simulink model "exemplo_bloco_Main"  (R2024b)
settings: Solver=ode45  StartTime=0.0  StopTime=200  RelTol=1e-6  EnableMultiTasking=on
settings Model: Creator=Mauricio  LastModifiedBy=johne
settings SolverCC: AlgebraicLoopSolver=TrustRegion
settings DataIOCC: LimitDataPoints=on  SaveFormat=Array  ReturnWorkspaceOutputs=off
settings OptimizationCC: LifeSpan=inf
settings DebuggingCC: SolverPrmCheckMsg=warning  UnconnectedInputMsg=warning  UnconnectedOutputMsg=warning  UnconnectedLineMsg=warning  SFUnexpectedBacktrackingDiag=warning  SFNoUnconditionalDefaultTransitionDiag=warning  SFExecutionAtInitializationDiag=none  ArithmeticOperatorsInVariantConditions=warning
settings HardwareCC: ProdBitPerPointer=32  ProdBitPerSizeT=32  ProdBitPerPtrDiffT=32  ProdLargestAtomicFloat=None  ProdIntDivRoundTo=Undefined  ProdEndianess=Unspecified  ProdWordSize=32  ProdHWDeviceType=32-bit Generic
settings ModelReferenceCC: EnableRefExpFcnMdlSchedulingChecks=on  PropagateSignalLabelsOutOfModel=off
settings SFSimCC: SimUseLocalCustomCode=off  CustomCodeUndefinedFunction=UseInterfaceOnly
settings RTWCC: RTWUseLocalCustomCode=off  GPUComputeCapability=3.5
settings CodeAppCC: StateflowObjectComments=on
settings GRTTargetCC: TargetLangStandard=C89/C90 (ANSI)
settings ConfigComp: CovMetricSettings=dw  CovSaveCumulativeToWorkspaceVar=on  CovSaveSingleToWorkspaceVar=on  CovExternalEMLEnable=off  CovSFcnEnable=off

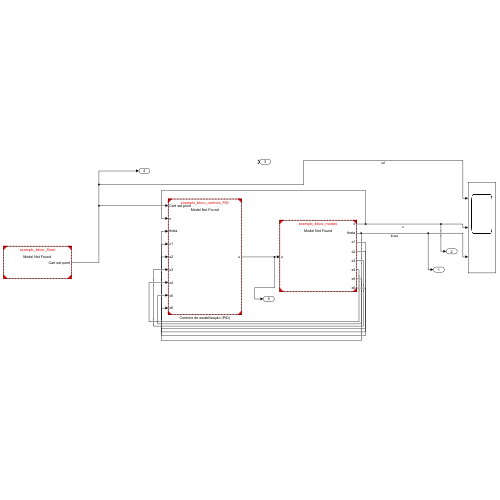
[thumbnail: Simulink's stored preview of the top-level diagram]
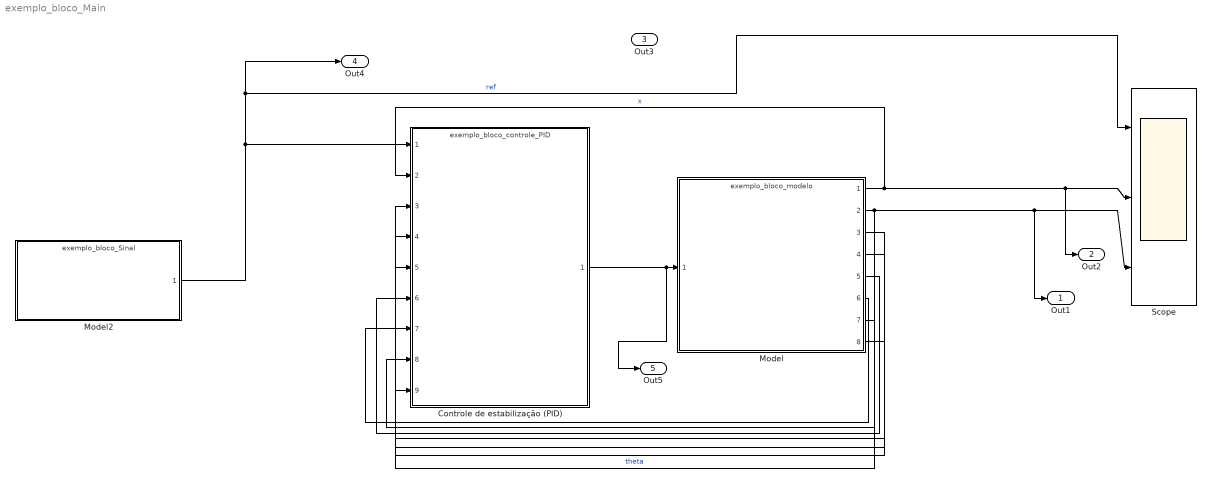
== system exemplo_bloco_Main ==
  Controle de estabilização (PID) : ModelReference  ModelNameDialog=exemplo_bloco_controle_PID.slx  SimulationMode=Normal  ModelReferenceVersion=12.70
  Model : ModelReference  ModelNameDialog=exemplo_bloco_modelo.slx  SimulationMode=Normal  ModelReferenceVersion=12.38
  Model2 : ModelReference  ModelNameDialog=exemplo_bloco_Sinal.slx  SimulationMode=Normal  ModelReferenceVersion=12.11
  Scope : Scope  NumInputPorts=3
  Out1 : Outport  VectorParamsAs1DForOutWhenUnconnected=off
  Out2 : Outport  Port=2  VectorParamsAs1DForOutWhenUnconnected=off
  Out3 : Outport  Port=3  VectorParamsAs1DForOutWhenUnconnected=off
  Out4 : Outport  Port=4  VectorParamsAs1DForOutWhenUnconnected=off
  Out5 : Outport  Port=5  VectorParamsAs1DForOutWhenUnconnected=off
  wires:
  Model2/1 -> Controle de estabilização (PID)/1, Out4/1, Scope/1  "ref"
  Controle de estabilização (PID)/1 -> Out5/1, Model/1
  Model/8 -> Controle de estabilização (PID)/9
  Model/7 -> Controle de estabilização (PID)/8
  Model/6 -> Controle de estabilização (PID)/7
  Model/5 -> Controle de estabilização (PID)/6
  Model/4 -> Controle de estabilização (PID)/5
  Model/3 -> Controle de estabilização (PID)/4
  Model/2 -> Controle de estabilização (PID)/3, Out1/1, Scope/3  "theta"
  Model/1 -> Controle de estabilização (PID)/2, Out2/1, Scope/2  "x"
